simulink model "Focault_Pendulum"  (R2020b)
settings: Solver=VariableStepAuto  StartTime=0.0  StopTime=10.0  RelTol=1e-3
model workspace (MAT data in the model file):
  g = 9.81
  l = 1
  lambda = 0.446699568755
  w = 7.27e-05
settings Model: Creator=Mrudul  LastModifiedBy=Mrudul

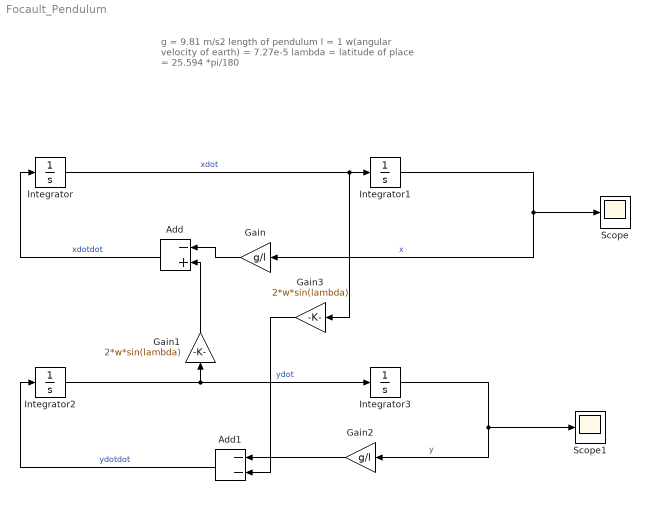
== system Focault_Pendulum ==
  note: g = 9.81 m/s2
      | length of pendulum l = 1
      | w(angular velocity of earth) = 7.27e-5
      | lambda = latitude of place = 25.594 *pi/180
  Add : Sum  Inputs=-+
  Add1 : Sum  Inputs=--
  Gain : Gain  Gain=g/l
  Gain1 : Gain  Gain=2*w*sin(lambda)
  Gain2 : Gain  Gain=g/l
  Gain3 : Gain  Gain=2*w*sin(lambda)
  Integrator : Integrator
  Integrator1 : Integrator  InitialCondition=0.005
  Integrator2 : Integrator
  Integrator3 : Integrator
  Scope : Scope
  Scope1 : Scope
  wires:
  Integrator/1 -> Gain3/1, Integrator1/1  "xdot"
  Add/1 -> Integrator/1  "xdotdot"
  Integrator1/1 -> Scope/1, Gain/1  "x"
  Integrator2/1 -> Gain1/1, Integrator3/1  "ydot"
  Add1/1 -> Integrator2/1  "ydotdot"
  Gain/1 -> Add/1
  Gain1/1 -> Add/2
  Integrator3/1 -> Gain2/1, Scope1/1  "y"
  Gain2/1 -> Add1/1
  Gain3/1 -> Add1/2
